simulink model "Fig277"  (R2014b)
settings: Solver=ode3  StartTime=0.0  StopTime=1  FixedStep=2e-5  RelTol=1e-5
libraries: commchan3 x1, dsparch4 x1, commrandsrc2 x1
settings Model: Creator=Dennis Silage  LastModifiedBy=Silage
settings DataIOCC: SignalLoggingSaveFormat=ModelDataLogs
settings OptimizationCC: ExpressionDepthLimit=2147483647  InitFltsAndDblsToZero=on
settings DebuggingCC: UnderspecifiedInitializationDetection=Classic  MergeDetectMultiDrivingBlocksExec=none  SolverPrmCheckMsg=none  FcnCallInpInsideContextMsg=UseLocalSettings  StateNameClashWarn=warning
settings GRTTargetCC: CombineOutputUpdateFcns=off  GRTInterface=on

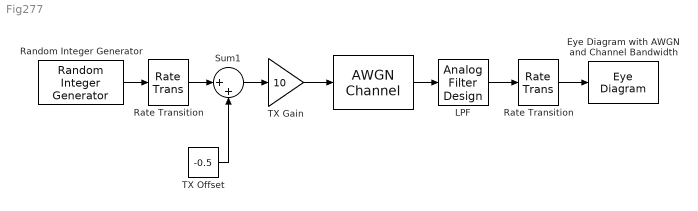
== system Fig277 ==
  "  " : commchan3/AWGN Channel  InputProcessing=Columns as channels (frame based)  seed=67  noiseMode=Variance from mask  EbNodB=16.98  EsNodB=10  SNRdB=50  bitsPerSym=1  Ps=25  Tsym=1e-3  variance=10.5
  Eye Diagram with AWGN and Channel Bandwidth : EyeDiagram  Tag=EyeDiagram
  LPF : dsparch4/Analog Filter Design  method=Chebyshev I  filttype=Lowpass  N=9  Wlo=2*pi*1200  Whi=80  Rp=0.1  Rs=40
  Random Integer Generator : commrandsrc2/Random Integer Generator  mul=2  seed=randseed  Ts=1e-3  frameBased=off  sampPerFrame=50  orient=on  outDataType=double
  Rate Transition : RateTransition  OutPortSampleTime=2e-5
  "Rate Transition " : RateTransition  OutPortSampleTime=2e-5
  Sum1 : Sum  Inputs=|++
  TX Gain : Gain  Gain=10
  TX Offset : Constant  Value=-0.5
  wires:
  Random Integer Generator/1 -> Rate Transition/1
  Rate Transition/1 -> Sum1/1
  Sum1/1 -> TX Gain/1
  TX Offset/1 -> Sum1/2
  "Rate Transition "/1 -> Eye Diagram with AWGN and Channel Bandwidth/1
  LPF/1 -> "Rate Transition "/1
  TX Gain/1 -> "  "/1
  "  "/1 -> LPF/1
